simulink model "nmm2DFullBody"  (R2015b)
settings: Solver=ode23s  StartTime=0.0  StopTime=13  FixedStep=1e-3  MaxStep=ts_max  RelTol=1e-3  AbsTol=1e-4
InitFcn:
  | addpath('../lib');
  | addpath('./init_script');
  | nms_model_MechInit
  | nms_model_ControlInit
StopFcn:
  | mRFX = struct;
  | 
  | mRFX.RStance = DataFromModel.Data(:,2)
  | mRFX.RGRF_AP = DataFromModel.Data(:,24)
  | mRFX.RGRF_VT = DataFromModel.Data(:,22)
  | mRFX.RAnkleAngle = DataFromModel.Data(:,8)
  | mRFX.RKneeAngle = DataFromModel.Data(:,7)
  | mRFX.RHipAngle = DataFromModel.Data(:,6)
  | mRFX.RAnkleTorque = DataFromModel.Data(:,20)
  | mRFX.RKneeTorque = DataFromModel.Data(:,19)
  | mRFX.RHipTorque = DataFromModel.Data(:,18)
  | 
  | mRFX.RMuscleGLU = DataFromModel.Data(:,32)
  | mRFX.RMuscleHF = DataFromModel.Data(:,33)
  | mRFX.RMuscleHAM = DataFromModel.Data(:,34)
  | mRFX.RMuscleVAS = DataFromModel.Data(:,35)
  | mRFX.RMuscleGAS = DataFromModel.Data(:,36)
  | mRFX.RMuscleSOL = DataFromModel.Data(:,37)
  | mRFX.RMuscleTA = DataFromModel.Data(:,38)
  | 
  | mRFX.LStance = DataFromModel.Data(:,1)
  | mRFX.LGRF_AP = DataFromModel.Data(:,23)
  | mRFX.LGRF_VT = DataFromModel.Data(:,21)
  | mRFX.LAnkleAngle = DataFromModel.Data(:,5)
  | mRFX.LKneeAngle = DataFromModel.Data(:,4)
  | mRFX.LHipAngle = DataFromModel.Data(:,3)
  | mRFX.LAnkleTorque = DataFromModel.Data(:,17)
  | mRFX.LKneeTorque = DataFromModel.Data(:,16)
  | mRFX.LHipTorque = DataFromModel.Data(:,15)
  | 
  | mRFX.LMuscleGLU = DataFromModel.Data(:,25)
  | mRFX.LMuscleHF = DataFromModel.Data(:,26)
  | mRFX.LMuscleHAM = DataFromModel.Data(:,27)
  | mRFX.LMuscleVAS = DataFromModel.Data(:,28)
  | mRFX.LMuscleGAS = DataFromModel.Data(:,29)
  | mRFX.LMuscleSOL = DataFromModel.Data(:,30)
  | mRFX.LMuscleTA = DataFromModel.Data(:,31)
values from neighbouring files (symbols this model uses):
  c = load('struct_mRFX_HAM_symetric_feedback.mat')    [Ex2b.m]
undefined symbols (not defined in the file or in its folder): alphaFmGas, alphaFmGlu, alphaFmHam, alphaFmSol, alphaFmVas, alphaLceHam, alphaLceHfl, alphaLceTa, alphaLceTa1, Amp, amp_var, c_jointstop, D12_F, D12_S, D12_T, D13_F, D1G_F, D1G_HAT, D1G_S, D1G_T, DeltaThRef, eref, FmaxGAS, FmaxGLU, FmaxHAM, FmaxHFL, FmaxSOL, FmaxTA, FmaxVAS, freq, freq_var, GainDeltaTheta, GainGAS, GainGLU, GainHAM, GainHAMHFL, GainHFL, GainKneOverExt, GainSOL, GainSOLTA, GainTA, GainVAS, In_F, In_HAT, In_S, In_T, K, k_gx, k_gy, k_pressure, K_swing, LceOffsetHAM, LceOffsetHFL, LceOffsetTA, LongDelay, loptGAS, loptGLU, loptHAM, loptHFL, loptSOL ... (+82)
libraries: nmc x77, mblibv1 x60, simulink x33, simulink_extras x18
(part 3 of 8)

== system nmm2DFullBody/Body Mechanics Layer (from Geyer s 2010 model)/Left Heel Contact/Ground Friction Model ==
  note: Vertical Ground Stiction Model
  note: Horizontal Ground Friction Model
  dy [m] : Inport
  vy [m/s] : Inport  Port=2
  x [m] : Inport  Port=3
  vx [m/s] : Inport  Port=4
  Contact! : EnablePort  StatesWhenEnabling=reset
  Data Type Conversion : DataTypeConversion  OutDataTypeStr=double
  Friction Switch : Subsystem
  Gain3 : Gain  Gain=k_gy
  Gain4 : Gain  Gain=1/v_gy_max
  Logical Operator : Logic  Operator=NOT  AllPortsSameDT=off  OutDataTypeStr=boolean
  Mux1 : Mux  Inputs=2
  Sum1 : Sum
  X-Axis Kinetic Friction Model : Subsystem
  X-Axis Static Friction Model : Subsystem
  Y-Axis Ground Force : Fcn  Expr="- u(1)  *  (1-u(2)) * (u(2)<1)"
  Fy_Ground[N] : Outport  OutputWhenDisabled=reset  InitialOutput=0
      settings: AttributesFormatString=initial = '%<InitialOutput>'\nwhen disabled = '%<OutputWhenDisabled>'
  Fx_Friction [N] : Outport  Port=2  OutputWhenDisabled=reset  InitialOutput=0
      settings: AttributesFormatString=initial = '%<InitialOutput>'\nwhen\ndisabled\n'%<OutputWhenDisabled>'
  Stiction! : Outport  Port=3  OutputWhenDisabled=reset  InitialOutput=0
      settings: AttributesFormatString=initial = '%<InitialOutput>'\nwhen\ndisabled\n'%<OutputWhenDisabled>'
  wires:
  Gain4/1 -> Mux1/2
  Gain3/1 -> Mux1/1
  Mux1/1 -> Y-Axis Ground Force/1
  Data Type Conversion/1 -> Stiction!/1
  Logical Operator/1 -> X-Axis Kinetic Friction Model/Enable
  X-Axis Kinetic Friction Model/2(Stiction!) -> Friction Switch/2(Stick!)
  X-Axis Static Friction Model/2(Sliding!) -> Friction Switch/1(Slide!)
  Friction Switch/1(Stiction) -> Data Type Conversion/1, Logical Operator/1, X-Axis Static Friction Model/Enable
  Sum1/1 -> Fx_Friction [N]/1
  X-Axis Static Friction Model/1(F_Stick [N]) -> Sum1/1
  X-Axis Kinetic Friction Model/3(F_Slide [N]) -> Sum1/2
  X-Axis Kinetic Friction Model/1(posFP [m]) -> X-Axis Static Friction Model/4(posFP [m])
  vx [m/s]/1 -> X-Axis Kinetic Friction Model/2(vel [m/s]), X-Axis Static Friction Model/3(vel [m/s])
  x [m]/1 -> X-Axis Kinetic Friction Model/1(pos [m]), X-Axis Static Friction Model/2(pos [m])
  vy [m/s]/1 -> Gain4/1
  dy [m]/1 -> Gain3/1
  Y-Axis Ground Force/1 -> Fy_Ground[N]/1, X-Axis Kinetic Friction Model/3(F_Normal [N]), X-Axis Static Friction Model/1(F_Normal [N])

== system nmm2DFullBody/Body Mechanics Layer (from Geyer s 2010 model)/Right Ball Contact/Ground Friction Model ==
  note: Horizontal Ground Friction Model
  note: Vertical Ground Stiction Model
  dy [m] : Inport
  vy [m/s] : Inport  Port=2
  x [m] : Inport  Port=3
  vx [m/s] : Inport  Port=4
  Contact! : EnablePort  StatesWhenEnabling=reset
  Data Type Conversion : DataTypeConversion  OutDataTypeStr=double
  Friction Switch : Subsystem
  Gain3 : Gain  Gain=k_gy
  Gain4 : Gain  Gain=1/v_gy_max
  Logical Operator : Logic  Operator=NOT  AllPortsSameDT=off  OutDataTypeStr=boolean
  Mux1 : Mux  Inputs=2
  Sum1 : Sum
  X-Axis Kinetic Friction Model : Subsystem
  X-Axis Static Friction Model : Subsystem
  Y-Axis Ground Force : Fcn  Expr="- u(1)  *  (1-u(2)) * (u(2)<1)"
  Fy_Ground[N] : Outport  OutputWhenDisabled=reset  InitialOutput=0
      settings: AttributesFormatString=initial = '%<InitialOutput>'\nwhen disabled = '%<OutputWhenDisabled>'
  Fx_Friction [N] : Outport  Port=2  OutputWhenDisabled=reset  InitialOutput=0
      settings: AttributesFormatString=initial = '%<InitialOutput>'\nwhen\ndisabled\n'%<OutputWhenDisabled>'
  Stiction! : Outport  Port=3  OutputWhenDisabled=reset  InitialOutput=0
      settings: AttributesFormatString=initial = '%<InitialOutput>'\nwhen\ndisabled\n'%<OutputWhenDisabled>'
  wires:
  dy [m]/1 -> Gain3/1
  vy [m/s]/1 -> Gain4/1
  x [m]/1 -> X-Axis Static Friction Model/2(pos [m]), X-Axis Kinetic Friction Model/1(pos [m])
  vx [m/s]/1 -> X-Axis Static Friction Model/3(vel [m/s]), X-Axis Kinetic Friction Model/2(vel [m/s])
  X-Axis Kinetic Friction Model/1(posFP [m]) -> X-Axis Static Friction Model/4(posFP [m])
  X-Axis Kinetic Friction Model/3(F_Slide [N]) -> Sum1/2
  X-Axis Static Friction Model/1(F_Stick [N]) -> Sum1/1
  Sum1/1 -> Fx_Friction [N]/1
  Friction Switch/1(Stiction) -> X-Axis Static Friction Model/Enable, Logical Operator/1, Data Type Conversion/1
  X-Axis Static Friction Model/2(Sliding!) -> Friction Switch/1(Slide!)
  X-Axis Kinetic Friction Model/2(Stiction!) -> Friction Switch/2(Stick!)
  Logical Operator/1 -> X-Axis Kinetic Friction Model/Enable
  Data Type Conversion/1 -> Stiction!/1
  Mux1/1 -> Y-Axis Ground Force/1
  Gain3/1 -> Mux1/1
  Gain4/1 -> Mux1/2
  Y-Axis Ground Force/1 -> Fy_Ground[N]/1, X-Axis Static Friction Model/1(F_Normal [N]), X-Axis Kinetic Friction Model/3(F_Normal [N])

== system nmm2DFullBody/Body Mechanics Layer (from Geyer s 2010 model)/Right Heel Contact/Ground Friction Model ==
  note: Vertical Ground Stiction Model
  note: Horizontal Ground Friction Model
  dy [m] : Inport
  vy [m/s] : Inport  Port=2
  x [m] : Inport  Port=3
  vx [m/s] : Inport  Port=4
  Contact! : EnablePort  StatesWhenEnabling=reset
  Data Type Conversion : DataTypeConversion  OutDataTypeStr=double
  Friction Switch : Subsystem
  Gain3 : Gain  Gain=k_gy
  Gain4 : Gain  Gain=1/v_gy_max
  Logical Operator : Logic  Operator=NOT  AllPortsSameDT=off  OutDataTypeStr=boolean
  Mux1 : Mux  Inputs=2
  Sum1 : Sum
  X-Axis Kinetic Friction Model : Subsystem
  X-Axis Static Friction Model : Subsystem
  Y-Axis Ground Force : Fcn  Expr="- u(1)  *  (1-u(2)) * (u(2)<1)"
  Fy_Ground[N] : Outport  OutputWhenDisabled=reset  InitialOutput=0
      settings: AttributesFormatString=initial = '%<InitialOutput>'\nwhen disabled = '%<OutputWhenDisabled>'
  Fx_Friction [N] : Outport  Port=2  OutputWhenDisabled=reset  InitialOutput=0
      settings: AttributesFormatString=initial = '%<InitialOutput>'\nwhen\ndisabled\n'%<OutputWhenDisabled>'
  Stiction! : Outport  Port=3  OutputWhenDisabled=reset  InitialOutput=0
      settings: AttributesFormatString=initial = '%<InitialOutput>'\nwhen\ndisabled\n'%<OutputWhenDisabled>'
  wires:
  Gain4/1 -> Mux1/2
  Gain3/1 -> Mux1/1
  Mux1/1 -> Y-Axis Ground Force/1
  Data Type Conversion/1 -> Stiction!/1
  Logical Operator/1 -> X-Axis Kinetic Friction Model/Enable
  X-Axis Kinetic Friction Model/2(Stiction!) -> Friction Switch/2(Stick!)
  X-Axis Static Friction Model/2(Sliding!) -> Friction Switch/1(Slide!)
  Friction Switch/1(Stiction) -> Data Type Conversion/1, Logical Operator/1, X-Axis Static Friction Model/Enable
  Sum1/1 -> Fx_Friction [N]/1
  X-Axis Static Friction Model/1(F_Stick [N]) -> Sum1/1
  X-Axis Kinetic Friction Model/3(F_Slide [N]) -> Sum1/2
  X-Axis Kinetic Friction Model/1(posFP [m]) -> X-Axis Static Friction Model/4(posFP [m])
  vx [m/s]/1 -> X-Axis Kinetic Friction Model/2(vel [m/s]), X-Axis Static Friction Model/3(vel [m/s])
  x [m]/1 -> X-Axis Kinetic Friction Model/1(pos [m]), X-Axis Static Friction Model/2(pos [m])
  vy [m/s]/1 -> Gain4/1
  dy [m]/1 -> Gain3/1
  Y-Axis Ground Force/1 -> Fy_Ground[N]/1, X-Axis Kinetic Friction Model/3(F_Normal [N]), X-Axis Static Friction Model/1(F_Normal [N])

== system nmm2DFullBody/Full Body Control (created using the nmc library)/Left Side/AnkleJoint left ==
  note: Ankle Joint
  phidphiAnkle : Inport
  PreTauAnkle : Inport  Port=2
  " Ankle Joint Limits" : Subsystem
  Demux : Demux  Outputs=2
  GotoDisabler_Component : nmc/GotoDisabler_Component  GotoTag=DisableNMC_JointLimits
  Sum : Sum  Inputs=|++
  Sum of Elements : Sum  Inputs=+
  TauAnkle : Outport
  wires:
  Demux/1 -> " Ankle Joint Limits"/1(phi [rad])
  Demux/2 -> " Ankle Joint Limits"/2(dphi [rad/s])
  PreTauAnkle/1 -> Sum of Elements/1
  phidphiAnkle/1 -> Demux/1
  " Ankle Joint Limits"/1(M_stop [Nm]) -> GotoDisabler_Component/1
  Sum/1 -> TauAnkle/1
  Sum of Elements/1 -> Sum/2
  GotoDisabler_Component/1 -> Sum/1

== system nmm2DFullBody/Full Body Control (created using the nmc library)/Left Side/GAS Muscle ==
  note: GAS Muscle
  phiKnee : Inport
  phiAnkle : Inport  Port=2
  StanceSwing : Inport  Port=3
  "GAS Actuation " : Subsystem
  GAS Control : Subsystem
  LOG_GasAnkle : Concatenate  NumInputs=1
  LOG_TauGasKnee : Concatenate  NumInputs=1
  StimGAS : ToWorkspace  VariableName=StimGASL  SaveFormat=Timeseries  SampleTime=-1
  TauGasKnee : Outport
  TauGasAnkle : Outport  Port=2
  wires:
  LOG_GasAnkle/1 -> TauGasAnkle/1
  LOG_TauGasKnee/1 -> TauGasKnee/1
  phiAnkle/1 -> "GAS Actuation "/2(phiAnkle)
  "GAS Actuation "/1(TauGasKnee) -> LOG_TauGasKnee/1
  "GAS Actuation "/2(TauGasAnkle) -> LOG_GasAnkle/1
  "GAS Actuation "/3(FmGas) -> GAS Control/1(FmGAS)
  StanceSwing/1 -> GAS Control/2(StanceSwing)
  phiKnee/1 -> "GAS Actuation "/1(phiKnee)
  GAS Control/1(StimGAS) -> StimGAS/1, "GAS Actuation "/3(StimGas)

== system nmm2DFullBody/Full Body Control (created using the nmc library)/Left Side/GLU Muscle ==
  note: GLU Muscle
  phiHip : Inport
  CLdxThigh : Inport  Port=2
  OLonCL : Inport  Port=3
  StanceSwing : Inport  Port=4
  GLU Actuation : Subsystem
  GLU Control : Subsystem
  LOG_TauGlu : Concatenate  NumInputs=1
  StimGLU : ToWorkspace  VariableName=StimGLU1  SaveFormat=Timeseries  SampleTime=-1
  TauGlu : Outport
  wires:
  LOG_TauGlu/1 -> TauGlu/1
  GLU Control/1(StimGlu) -> GLU Actuation/2(StimGlu), StimGLU/1
  GLU Actuation/2(FmGlu) -> GLU Control/1(FmGlu)
  OLonCL/1 -> GLU Control/5(OLonCL)
  [ThetaDelayed] -> GLU Control/2(Theta)
  [dThetaDelayed] -> GLU Control/3(dTheta)
  phiHip/1 -> GLU Actuation/1(phiHip)
  CLdxThigh/1 -> GLU Control/4(CLdxThigh)
  StanceSwing/1 -> GLU Control/6(StanceSwing)
  GLU Actuation/1(TauGlu) -> LOG_TauGlu/1

== system nmm2DFullBody/Full Body Control (created using the nmc library)/Left Side/HFL&HAM Muscles ==
  note: HFL&HAM Muscles
  phiHip : Inport
  phiKnee : Inport  Port=2
  CLdxThigh : Inport  Port=3
  OLonCL : Inport  Port=4
  StanceSwing : Inport  Port=5
  "HAM Actuation " : Subsystem
  HFL Actuation : Subsystem
  HFL&HAM Control : Subsystem
  LOG_TauHFL : Concatenate  NumInputs=1
  LOG_TauHamHip : Concatenate  NumInputs=1
  LOG_TauHamKnee : Concatenate  NumInputs=1
  StimHAM : ToWorkspace  VariableName=StimHAM  SaveFormat=Timeseries  SampleTime=-1
  StimHFL : ToWorkspace  VariableName=StimHFL  SaveFormat=Timeseries  SampleTime=-1
  TauHFL : Outport
  TauHamHip : Outport  Port=2
  TauHamKnee : Outport  Port=3
  wires:
  LOG_TauHamKnee/1 -> TauHamKnee/1
  LOG_TauHamHip/1 -> TauHamHip/1
  LOG_TauHFL/1 -> TauHFL/1
  HFL&HAM Control/2(StimHAM) -> StimHAM/1, "HAM Actuation "/3(StimHam)
  StanceSwing/1 -> HFL&HAM Control/8(StanceSwing)
  [dThetaDelayed] -> HFL&HAM Control/5(dTheta)
  [ThetaDelayed] -> HFL&HAM Control/4(Theta)
  phiKnee/1 -> "HAM Actuation "/2(phiKnee)
  HFL Actuation/1(TauHFL) -> LOG_TauHFL/1
  CLdxThigh/1 -> HFL&HAM Control/6(CLdxThigh)
  "HAM Actuation "/2(TauHamKnee) -> LOG_TauHamKnee/1
  phiHip/1 -> "HAM Actuation "/1(phiHip), HFL Actuation/1(phiHip)
  "HAM Actuation "/1(TauHamHip) -> LOG_TauHamHip/1
  OLonCL/1 -> HFL&HAM Control/7(OLonCL)
  HFL Actuation/2(LceHFL) -> HFL&HAM Control/1(LceHFL)
  "HAM Actuation "/4(FmHam) -> HFL&HAM Control/3(FmHam)
  "HAM Actuation "/3(LceHam) -> HFL&HAM Control/2(LceHam)
  HFL&HAM Control/1(StimHFL) -> StimHFL/1, HFL Actuation/2(StimHFL)

== system nmm2DFullBody/Full Body Control (created using the nmc library)/Left Side/HipJoint left ==
  note: Hip Joint
  phidphiHip : Inport
  PreTauHip : Inport  Port=2
  Demux2 : Demux  Outputs=2
  GotoDisabler_Component : nmc/GotoDisabler_Component  GotoTag=DisableNMC_JointLimits
  Hip Joint Limits : Subsystem
  Sum of Elements : Sum  Inputs=+
  Sum16 : Sum  Inputs=|++
  TauHip : Outport
  wires:
  phidphiHip/1 -> Demux2/1
  Demux2/1 -> Hip Joint Limits/1(phi [rad])
  Demux2/2 -> Hip Joint Limits/2(dphi [rad/s])
  Sum16/1 -> TauHip/1
  PreTauHip/1 -> Sum of Elements/1
  Sum of Elements/1 -> Sum16/2
  Hip Joint Limits/1(M_stop [Nm]) -> GotoDisabler_Component/1
  GotoDisabler_Component/1 -> Sum16/1

== system nmm2DFullBody/Full Body Control (created using the nmc library)/Left Side/KneeJoint left ==
  note: Knee Joint
  phidphiKnee : Inport
  PreTauKnee : Inport  Port=2
  Demux1 : Demux  Outputs=2
  Gain : Gain  Gain=-1
  GotoDisabler_Component : nmc/GotoDisabler_Component  GotoTag=DisableNMC_JointLimits
  Knee Joint Limits : Subsystem
  Sum : Sum  Inputs=|++
  Sum of Elements : Sum  Inputs=+
  TauKnee : Outport
  wires:
  Demux1/1 -> Knee Joint Limits/1(phi [rad])
  Demux1/2 -> Knee Joint Limits/2(dphi [rad/s])
  phidphiKnee/1 -> Demux1/1
  Sum/1 -> TauKnee/1
  PreTauKnee/1 -> Sum of Elements/1
  Sum of Elements/1 -> Gain/1
  Gain/1 -> Sum/2
  Knee Joint Limits/1(M_stop [Nm]) -> GotoDisabler_Component/1
  GotoDisabler_Component/1 -> Sum/1

== system nmm2DFullBody/Full Body Control (created using the nmc library)/Left Side/SOL&TA Muscles ==
  note: SOL&TA Muscles
  phiAnkle : Inport
  StanceSwing : Inport  Port=2
  LOG_StimSOL : Concatenate  NumInputs=1
  LOG_StimTA : Concatenate  NumInputs=1
  LOG_TauSOL : Concatenate  NumInputs=1
  LOG_TauTA : Concatenate  NumInputs=1
  SOL Actuation : Subsystem
  SOL&TA Control : Subsystem
  StimSOL : ToWorkspace  VariableName=StimSOLL  SaveFormat=Timeseries  SampleTime=-1
  StimTA : ToWorkspace  VariableName=StimTAL  SaveFormat=Timeseries  SampleTime=-1
  TA Actuation : Subsystem
  TauTA : Outport
  TauSOL : Outport  Port=2
  wires:
  LOG_StimSOL/1 -> StimSOL/1, SOL Actuation/2(StimSOL)
  LOG_StimTA/1 -> TA Actuation/2(StimTA), StimTA/1
  LOG_TauSOL/1 -> TauSOL/1
  LOG_TauTA/1 -> TauTA/1
  TA Actuation/2(TauTa) -> LOG_TauTA/1
  phiAnkle/1 -> SOL Actuation/1(phiAnkle), TA Actuation/1(phiAnkle)
  TA Actuation/1(LceTA) -> SOL&TA Control/1(LceTA)
  StanceSwing/1 -> SOL&TA Control/3(StanceSwing)
  SOL&TA Control/1(StimTA) -> LOG_StimTA/1
  SOL Actuation/1(TauSOL) -> LOG_TauSOL/1
  SOL Actuation/2(FmSOL) -> SOL&TA Control/2(FmSOL)
  SOL&TA Control/2(StimSOL) -> LOG_StimSOL/1

== system nmm2DFullBody/Full Body Control (created using the nmc library)/Left Side/VAS Muscle ==
  note: VAS Muscle
  phiKnee : Inport
  OLdxThigh : Inport  Port=2
  OLonCL : Inport  Port=3
  CLKneeState : Inport  Port=4
  StanceSwing : Inport  Port=5
  LOG_TauVas : Concatenate  NumInputs=1
  StimVAS : ToWorkspace  VariableName=StimVAS  SaveFormat=Timeseries  SampleTime=-1
  "VAS Actuation " : Subsystem
  VAS Control : Subsystem
  TauVas : Outport
  wires:
  LOG_TauVas/1 -> TauVas/1
  VAS Control/1(StimVAS) -> StimVAS/1, "VAS Actuation "/2(StimVas)
  "VAS Actuation "/2(FmVas) -> VAS Control/1(FmVAS)
  "VAS Actuation "/1(TauVas) -> LOG_TauVas/1
  OLonCL/1 -> VAS Control/3(OLonCL)
  StanceSwing/1 -> VAS Control/5(StanceSwing)
  OLdxThigh/1 -> VAS Control/2(OLdxThigh)
  phiKnee/1 -> "VAS Actuation "/1(phiKnee)
  CLKneeState/1 -> VAS Control/4(CLKneeState)

== system nmm2DFullBody/Full Body Control (created using the nmc library)/Right Side/GAS Muscle ==
  note: GAS Muscle
  phiKnee : Inport
  phiAnkle : Inport  Port=2
  StanceSwing : Inport  Port=3
  "GAS Actuation " : Subsystem
  GAS Control : Subsystem
  LOG_GasAnkle : Concatenate  NumInputs=1
  LOG_TauGasKnee : Concatenate  NumInputs=1
  StimGAS : ToWorkspace  VariableName=StimGASR  SaveFormat=Timeseries  SampleTime=-1
  TauGasKnee : Outport
  TauGasAnkle : Outport  Port=2
  wires:
  LOG_GasAnkle/1 -> TauGasAnkle/1
  LOG_TauGasKnee/1 -> TauGasKnee/1
  phiAnkle/1 -> "GAS Actuation "/2(phiAnkle)
  "GAS Actuation "/1(TauGasKnee) -> LOG_TauGasKnee/1
  "GAS Actuation "/2(TauGasAnkle) -> LOG_GasAnkle/1
  "GAS Actuation "/3(FmGas) -> GAS Control/1(FmGAS)
  StanceSwing/1 -> GAS Control/2(StanceSwing)
  phiKnee/1 -> "GAS Actuation "/1(phiKnee)
  GAS Control/1(StimGAS) -> StimGAS/1, "GAS Actuation "/3(StimGas)

== system nmm2DFullBody/Full Body Control (created using the nmc library)/Right Side/GLU Muscle ==
  note: GLU Muscle
  phiHip : Inport
  CLdxThigh : Inport  Port=2
  OLonCL : Inport  Port=3
  StanceSwing : Inport  Port=4
  GLU Actuation : Subsystem
  GLU Control : Subsystem
  LOG_TauGlu : Concatenate  NumInputs=1
  StimGLU : ToWorkspace  VariableName=StimGLUR  SaveFormat=Timeseries  SampleTime=-1
  TauGlu : Outport
  wires:
  LOG_TauGlu/1 -> TauGlu/1
  GLU Control/1(StimGlu) -> GLU Actuation/2(StimGlu), StimGLU/1
  GLU Actuation/2(FmGlu) -> GLU Control/1(FmGlu)
  OLonCL/1 -> GLU Control/5(OLonCL)
  [ThetaDelayed] -> GLU Control/2(Theta)
  [dThetaDelayed] -> GLU Control/3(dTheta)
  phiHip/1 -> GLU Actuation/1(phiHip)
  CLdxThigh/1 -> GLU Control/4(CLdxThigh)
  StanceSwing/1 -> GLU Control/6(StanceSwing)
  GLU Actuation/1(TauGlu) -> LOG_TauGlu/1

== system nmm2DFullBody/Full Body Control (created using the nmc library)/Right Side/HFL&HAM Muscles ==
  note: HFL&HAM Muscles
  phiHip : Inport
  phiKnee : Inport  Port=2
  CLdxThigh : Inport  Port=3
  OLonCL : Inport  Port=4
  StanceSwing : Inport  Port=5
  "HAM Actuation " : Subsystem
  HFL Actuation : Subsystem
  HFL&HAM Control : Subsystem
  LOG_TauHFL : Concatenate  NumInputs=1
  LOG_TauHamHip : Concatenate  NumInputs=1
  LOG_TauHamKnee : Concatenate  NumInputs=1
  StimHAM : ToWorkspace  VariableName=StimHAMR  SaveFormat=Timeseries  SampleTime=-1
  StimHFL : ToWorkspace  VariableName=StimHFLR  SaveFormat=Timeseries  SampleTime=-1
  TauHFL : Outport
  TauHamHip : Outport  Port=2
  TauHamKnee : Outport  Port=3
  wires:
  LOG_TauHamKnee/1 -> TauHamKnee/1
  LOG_TauHamHip/1 -> TauHamHip/1
  LOG_TauHFL/1 -> TauHFL/1
  HFL&HAM Control/2(StimHAM) -> StimHAM/1, "HAM Actuation "/3(StimHam)
  StanceSwing/1 -> HFL&HAM Control/8(StanceSwing)
  [dThetaDelayed] -> HFL&HAM Control/5(dTheta)
  [ThetaDelayed] -> HFL&HAM Control/4(Theta)
  phiKnee/1 -> "HAM Actuation "/2(phiKnee)
  HFL Actuation/1(TauHFL) -> LOG_TauHFL/1
  CLdxThigh/1 -> HFL&HAM Control/6(CLdxThigh)
  "HAM Actuation "/2(TauHamKnee) -> LOG_TauHamKnee/1
  phiHip/1 -> "HAM Actuation "/1(phiHip), HFL Actuation/1(phiHip)
  "HAM Actuation "/1(TauHamHip) -> LOG_TauHamHip/1
  OLonCL/1 -> HFL&HAM Control/7(OLonCL)
  HFL Actuation/2(LceHFL) -> HFL&HAM Control/1(LceHFL)
  "HAM Actuation "/4(FmHam) -> HFL&HAM Control/3(FmHam)
  "HAM Actuation "/3(LceHam) -> HFL&HAM Control/2(LceHam)
  HFL&HAM Control/1(StimHFL) -> StimHFL/1, HFL Actuation/2(StimHFL)

== system nmm2DFullBody/Full Body Control (created using the nmc library)/Right Side/SOL&TA Muscles ==
  note: SOL&TA Muscles
  phiAnkle : Inport
  StanceSwing : Inport  Port=2
  LOG_StimSOL : Concatenate  NumInputs=1
  LOG_StimTA : Concatenate  NumInputs=1
  LOG_TauSOL : Concatenate  NumInputs=1
  LOG_TauTA : Concatenate  NumInputs=1
  SOL Actuation : Subsystem
  SOL&TA Control : Subsystem
  StimSOL : ToWorkspace  VariableName=StimSOLR  SaveFormat=Timeseries  SampleTime=-1
  StimTA : ToWorkspace  VariableName=StimTAR  SaveFormat=Timeseries  SampleTime=-1
  TA Actuation : Subsystem
  TauTA : Outport
  TauSOL : Outport  Port=2
  wires:
  LOG_StimSOL/1 -> StimSOL/1, SOL Actuation/2(StimSOL)
  LOG_StimTA/1 -> TA Actuation/2(StimTA), StimTA/1
  LOG_TauSOL/1 -> TauSOL/1
  LOG_TauTA/1 -> TauTA/1
  TA Actuation/2(TauTa) -> LOG_TauTA/1
  phiAnkle/1 -> SOL Actuation/1(phiAnkle), TA Actuation/1(phiAnkle)
  TA Actuation/1(LceTA) -> SOL&TA Control/1(LceTA)
  StanceSwing/1 -> SOL&TA Control/3(StanceSwing)
  SOL&TA Control/1(StimTA) -> LOG_StimTA/1
  SOL Actuation/1(TauSOL) -> LOG_TauSOL/1
  SOL Actuation/2(FmSOL) -> SOL&TA Control/2(FmSOL)
  SOL&TA Control/2(StimSOL) -> LOG_StimSOL/1

== system nmm2DFullBody/Full Body Control (created using the nmc library)/Right Side/VAS Muscle ==
  note: VAS Muscle
  phiKnee : Inport
  OLdxThigh : Inport  Port=2
  OLonCL : Inport  Port=3
  CLKneeState : Inport  Port=4
  StanceSwing : Inport  Port=5
  LOG_TauVas : Concatenate  NumInputs=1
  StimVAS : ToWorkspace  VariableName=StimVASR  SaveFormat=Timeseries  SampleTime=-1
  "VAS Actuation " : Subsystem
  VAS Control : Subsystem
  TauVas : Outport
  wires:
  LOG_TauVas/1 -> TauVas/1
  VAS Control/1(StimVAS) -> StimVAS/1, "VAS Actuation "/2(StimVas)
  "VAS Actuation "/2(FmVas) -> VAS Control/1(FmVAS)
  "VAS Actuation "/1(TauVas) -> LOG_TauVas/1
  OLonCL/1 -> VAS Control/3(OLonCL)
  StanceSwing/1 -> VAS Control/5(StanceSwing)
  OLdxThigh/1 -> VAS Control/2(OLdxThigh)
  phiKnee/1 -> "VAS Actuation "/1(phiKnee)
  CLKneeState/1 -> VAS Control/4(CLKneeState)

== system nmm2DFullBody/Full Body Control (created using the nmc library)/Subsystem/Parameter variation ==
  Alpha variation : Subsystem  Commented=on
  Amplitude Variation : Subsystem  Commented=on
  Freq variation : Subsystem  Commented=on

== system nmm2DFullBody/Body Mechanics Layer (from Geyer s 2010 model)/Left Ball Contact/Ground Friction Model/Friction Switch ==
  note: Static/Kinetic Friction Switch
  Slide! : Inport
  Stick! : Inport  Port=2
  Memory : Memory
  S-R Flip-Flop : simulink_extras/Flip Flops/S-R Flip-Flop  initial_condition=1
  Terminator : Terminator
  Stiction : Outport
  wires:
  S-R Flip-Flop/1 -> Memory/1
  S-R Flip-Flop/2 -> Terminator/1
  Stick!/1 -> S-R Flip-Flop/1
  Slide!/1 -> S-R Flip-Flop/2
  Memory/1 -> Stiction/1

== system nmm2DFullBody/Body Mechanics Layer (from Geyer s 2010 model)/Left Ball Contact/Ground Friction Model/X-Axis Kinetic Friction Model ==
  note: Kinetic Friction Model
  note: Footpoint Determiner
  note: Sliding Limit Detector
  pos [m] : Inport
  vel [m/s] : Inport  Port=2
  F_Normal [N] : Inport  Port=3
  Enable : EnablePort  StatesWhenEnabling=reset  ZeroCross=off
  Abs : Abs
  Constant : Constant  Value=vLimit
  FixPt Relational Operator : RelationalOperator  Operator=>  OutDataTypeStr=boolean  ZeroCross=off
  Memory : Memory
  Negative : simulink/Logic and Bit Operations/Compare To Zero  relop=<  OutDataTypeStr=boolean
  Product : Product  RndMeth=Zero
  Sign1 : Signum
  Sum : Sum  Inputs=|+-
  reverse : Gain  Gain=-1
  sliding friction coefficient : Gain  Gain=mu_slide
  posFP [m] : Outport  InitialOutput=0
      settings: AttributesFormatString=initial = '%<InitialOutput>'\nwhen disabled = '%<OutputWhenDisabled>'
  Stiction! : Outport  Port=2  OutputWhenDisabled=reset  InitialOutput=0
      settings: AttributesFormatString=initial = '%<InitialOutput>'\nwhen disabled = '%<OutputWhenDisabled>'
  F_Slide [N] : Outport  Port=3  OutputWhenDisabled=reset  InitialOutput=0
      settings: AttributesFormatString=initial = '%<InitialOutput>'\nwhen disabled = '%<OutputWhenDisabled>'
  wires:
  reverse/1 -> Product/1
  F_Normal [N]/1 -> sliding friction coefficient/1
  vel [m/s]/1 -> Sign1/1, Abs/1
  pos [m]/1 -> posFP [m]/1
  Product/1 -> F_Slide [N]/1
  sliding friction coefficient/1 -> Product/2
  Sign1/1 -> reverse/1
  FixPt Relational Operator/1 -> Stiction!/1
  Memory/1 -> FixPt Relational Operator/2
  Negative/1 -> FixPt Relational Operator/1, Memory/1
  Abs/1 -> Sum/1
  Sum/1 -> Negative/1
  Constant/1 -> Sum/2

== system nmm2DFullBody/Body Mechanics Layer (from Geyer s 2010 model)/Left Ball Contact/Ground Friction Model/X-Axis Static Friction Model ==
  note: Stiction Limit Detector
  note: Static Friction Model
  note: Zero multiplication prevents
      | horizontal friction model from
      | oscillating between static and kinetic
      | friction when the vertical force is zero but
      | the ground level is not yet reached
      | in the upward motion
  F_Normal [N] : Inport
  pos [m] : Inport  Port=2
  vel [m/s] : Inport  Port=3
  posFP [m] : Inport  Port=4
  Enable : EnablePort  StatesWhenEnabling=reset  ZeroCross=off
  Abs : Abs
  Abs. : Abs
  Check Vertical Friction : Product  RndMeth=Zero
  FixPt Relational Operator : RelationalOperator  Operator=>  OutDataTypeStr=boolean  ZeroCross=off
  Gain3 : Gain  Gain=k_gx
  Gain4 : Gain  Gain=1/v_gx_max
  Memory : Memory
  Mux1 : Mux  Inputs=2
  Positive : simulink/Logic and Bit Operations/Compare To Zero  relop=>  OutDataTypeStr=boolean
  Positive1 : simulink/Logic and Bit Operations/Compare To Zero  relop=>  OutDataTypeStr=boolean
  Sum : Sum  Inputs=-+
  Sum2 : Sum  Inputs=-+|
  X-Axis Stiction Force : Fcn  Expr=-u(1) * (1+sgn(u(1))*u(2))
  stiction limit force : Gain  Gain=mu_stick
  F_Stick [N] : Outport  OutputWhenDisabled=reset  InitialOutput=0
      settings: AttributesFormatString=when disabled: %<OutputWhenDisabled>\ninitial: %<InitialOutput>
  Sliding! : Outport  Port=2  OutputWhenDisabled=reset  InitialOutput=0
      settings: AttributesFormatString=when disabled: %<OutputWhenDisabled>\ninitial: %<InitialOutput>
  wires:
  F_Normal [N]/1 -> stiction limit force/1, Positive1/1
  Sum2/1 -> Gain3/1  "dx"
  pos [m]/1 -> Sum2/2
  posFP [m]/1 -> Sum2/1
  vel [m/s]/1 -> Gain4/1
  Sum/1 -> Positive/1
  Memory/1 -> FixPt Relational Operator/2
  Positive/1 -> FixPt Relational Operator/1, Memory/1
  Abs./1 -> Sum/2
  Mux1/1 -> X-Axis Stiction Force/1
  Gain3/1 -> Mux1/1
  Gain4/1 -> Mux1/2
  FixPt Relational Operator/1 -> Sliding!/1
  Abs/1 -> Sum/1
  stiction limit force/1 -> Abs/1
  X-Axis Stiction Force/1 -> Check Vertical Friction/1
  Positive1/1 -> Check Vertical Friction/2
  Check Vertical Friction/1 -> F_Stick [N]/1, Abs./1

== system nmm2DFullBody/Body Mechanics Layer (from Geyer s 2010 model)/Left Heel Contact/Ground Friction Model/Friction Switch ==
  note: Static/Kinetic Friction Switch
  Slide! : Inport
  Stick! : Inport  Port=2
  Memory : Memory
  S-R Flip-Flop : simulink_extras/Flip Flops/S-R Flip-Flop  initial_condition=1
  Terminator : Terminator
  Stiction : Outport
  wires:
  Memory/1 -> Stiction/1
  Slide!/1 -> S-R Flip-Flop/2
  Stick!/1 -> S-R Flip-Flop/1
  S-R Flip-Flop/2 -> Terminator/1
  S-R Flip-Flop/1 -> Memory/1

== system nmm2DFullBody/Body Mechanics Layer (from Geyer s 2010 model)/Left Heel Contact/Ground Friction Model/X-Axis Kinetic Friction Model ==
  note: Sliding Limit Detector
  note: Footpoint Determiner
  note: Kinetic Friction Model
  pos [m] : Inport
  vel [m/s] : Inport  Port=2
  F_Normal [N] : Inport  Port=3
  Enable : EnablePort  StatesWhenEnabling=reset  ZeroCross=off
  Abs : Abs
  Constant : Constant  Value=vLimit
  FixPt Relational Operator : RelationalOperator  Operator=>  OutDataTypeStr=boolean  ZeroCross=off
  Memory : Memory
  Negative : simulink/Logic and Bit Operations/Compare To Zero  relop=<  OutDataTypeStr=boolean
  Product : Product  RndMeth=Zero
  Sign1 : Signum
  Sum : Sum  Inputs=|+-
  reverse : Gain  Gain=-1
  sliding friction coefficient : Gain  Gain=mu_slide
  posFP [m] : Outport  InitialOutput=0
      settings: AttributesFormatString=initial = '%<InitialOutput>'\nwhen disabled = '%<OutputWhenDisabled>'
  Stiction! : Outport  Port=2  OutputWhenDisabled=reset  InitialOutput=0
      settings: AttributesFormatString=initial = '%<InitialOutput>'\nwhen disabled = '%<OutputWhenDisabled>'
  F_Slide [N] : Outport  Port=3  OutputWhenDisabled=reset  InitialOutput=0
      settings: AttributesFormatString=initial = '%<InitialOutput>'\nwhen disabled = '%<OutputWhenDisabled>'
  wires:
  Constant/1 -> Sum/2
  Sum/1 -> Negative/1
  Abs/1 -> Sum/1
  Negative/1 -> Memory/1, FixPt Relational Operator/1
  Memory/1 -> FixPt Relational Operator/2
  FixPt Relational Operator/1 -> Stiction!/1
  Sign1/1 -> reverse/1
  sliding friction coefficient/1 -> Product/2
  Product/1 -> F_Slide [N]/1
  pos [m]/1 -> posFP [m]/1
  vel [m/s]/1 -> Abs/1, Sign1/1
  F_Normal [N]/1 -> sliding friction coefficient/1
  reverse/1 -> Product/1

== system nmm2DFullBody/Body Mechanics Layer (from Geyer s 2010 model)/Left Heel Contact/Ground Friction Model/X-Axis Static Friction Model ==
  note: Static Friction Model
  note: Stiction Limit Detector
  note: Zero multiplication prevents
      | horizontal friction model from
      | oscillating between static and kinetic
      | friction when the vertical force is zero but
      | the ground level is not yet reached
      | in the upward motion
  F_Normal [N] : Inport
  pos [m] : Inport  Port=2
  vel [m/s] : Inport  Port=3
  posFP [m] : Inport  Port=4
  Enable : EnablePort  StatesWhenEnabling=reset  ZeroCross=off
  Abs : Abs
  Abs. : Abs
  Check Vertical Friction : Product  RndMeth=Zero
  FixPt Relational Operator : RelationalOperator  Operator=>  OutDataTypeStr=boolean  ZeroCross=off
  Gain3 : Gain  Gain=k_gx
  Gain4 : Gain  Gain=1/v_gx_max
  Memory : Memory
  Mux1 : Mux  Inputs=2
  Positive : simulink/Logic and Bit Operations/Compare To Zero  relop=>  OutDataTypeStr=boolean
  Positive1 : simulink/Logic and Bit Operations/Compare To Zero  relop=>  OutDataTypeStr=boolean
  Sum : Sum  Inputs=-+
  Sum2 : Sum  Inputs=-+|
  X-Axis Stiction Force : Fcn  Expr=-u(1) * (1+sgn(u(1))*u(2))
  stiction limit force : Gain  Gain=mu_stick
  F_Stick [N] : Outport  OutputWhenDisabled=reset  InitialOutput=0
      settings: AttributesFormatString=when disabled: %<OutputWhenDisabled>\ninitial: %<InitialOutput>
  Sliding! : Outport  Port=2  OutputWhenDisabled=reset  InitialOutput=0
      settings: AttributesFormatString=when disabled: %<OutputWhenDisabled>\ninitial: %<InitialOutput>
  wires:
  F_Normal [N]/1 -> stiction limit force/1, Positive1/1
  Sum2/1 -> Gain3/1  "dx"
  pos [m]/1 -> Sum2/2
  posFP [m]/1 -> Sum2/1
  vel [m/s]/1 -> Gain4/1
  Sum/1 -> Positive/1
  Memory/1 -> FixPt Relational Operator/2
  Positive/1 -> FixPt Relational Operator/1, Memory/1
  Abs./1 -> Sum/2
  Mux1/1 -> X-Axis Stiction Force/1
  Gain3/1 -> Mux1/1
  Gain4/1 -> Mux1/2
  FixPt Relational Operator/1 -> Sliding!/1
  Abs/1 -> Sum/1
  stiction limit force/1 -> Abs/1
  X-Axis Stiction Force/1 -> Check Vertical Friction/1
  Positive1/1 -> Check Vertical Friction/2
  Check Vertical Friction/1 -> F_Stick [N]/1, Abs./1

== system nmm2DFullBody/Body Mechanics Layer (from Geyer s 2010 model)/Right Ball Contact/Ground Friction Model/Friction Switch ==
  note: Static/Kinetic Friction Switch
  Slide! : Inport
  Stick! : Inport  Port=2
  Memory : Memory
  S-R Flip-Flop : simulink_extras/Flip Flops/S-R Flip-Flop  initial_condition=1
  Terminator : Terminator
  Stiction : Outport
  wires:
  S-R Flip-Flop/1 -> Memory/1
  S-R Flip-Flop/2 -> Terminator/1
  Stick!/1 -> S-R Flip-Flop/1
  Slide!/1 -> S-R Flip-Flop/2
  Memory/1 -> Stiction/1

== system nmm2DFullBody/Body Mechanics Layer (from Geyer s 2010 model)/Right Ball Contact/Ground Friction Model/X-Axis Kinetic Friction Model ==
  note: Kinetic Friction Model
  note: Footpoint Determiner
  note: Sliding Limit Detector
  pos [m] : Inport
  vel [m/s] : Inport  Port=2
  F_Normal [N] : Inport  Port=3
  Enable : EnablePort  StatesWhenEnabling=reset  ZeroCross=off
  Abs : Abs
  Constant : Constant  Value=vLimit
  FixPt Relational Operator : RelationalOperator  Operator=>  OutDataTypeStr=boolean  ZeroCross=off
  Memory : Memory
  Negative : simulink/Logic and Bit Operations/Compare To Zero  relop=<  OutDataTypeStr=boolean
  Product : Product  RndMeth=Zero
  Sign1 : Signum
  Sum : Sum  Inputs=|+-
  reverse : Gain  Gain=-1
  sliding friction coefficient : Gain  Gain=mu_slide
  posFP [m] : Outport  InitialOutput=0
      settings: AttributesFormatString=initial = '%<InitialOutput>'\nwhen disabled = '%<OutputWhenDisabled>'
  Stiction! : Outport  Port=2  OutputWhenDisabled=reset  InitialOutput=0
      settings: AttributesFormatString=initial = '%<InitialOutput>'\nwhen disabled = '%<OutputWhenDisabled>'
  F_Slide [N] : Outport  Port=3  OutputWhenDisabled=reset  InitialOutput=0
      settings: AttributesFormatString=initial = '%<InitialOutput>'\nwhen disabled = '%<OutputWhenDisabled>'
  wires:
  reverse/1 -> Product/1
  F_Normal [N]/1 -> sliding friction coefficient/1
  vel [m/s]/1 -> Sign1/1, Abs/1
  pos [m]/1 -> posFP [m]/1
  Product/1 -> F_Slide [N]/1
  sliding friction coefficient/1 -> Product/2
  Sign1/1 -> reverse/1
  FixPt Relational Operator/1 -> Stiction!/1
  Memory/1 -> FixPt Relational Operator/2
  Negative/1 -> FixPt Relational Operator/1, Memory/1
  Abs/1 -> Sum/1
  Sum/1 -> Negative/1
  Constant/1 -> Sum/2

== system nmm2DFullBody/Body Mechanics Layer (from Geyer s 2010 model)/Right Ball Contact/Ground Friction Model/X-Axis Static Friction Model ==
  note: Stiction Limit Detector
  note: Static Friction Model
  note: Zero multiplication prevents
      | horizontal friction model from
      | oscillating between static and kinetic
      | friction when the vertical force is zero but
      | the ground level is not yet reached
      | in the upward motion
  F_Normal [N] : Inport
  pos [m] : Inport  Port=2
  vel [m/s] : Inport  Port=3
  posFP [m] : Inport  Port=4
  Enable : EnablePort  StatesWhenEnabling=reset  ZeroCross=off
  Abs : Abs
  Abs. : Abs
  Check Vertical Friction : Product  RndMeth=Zero
  FixPt Relational Operator : RelationalOperator  Operator=>  OutDataTypeStr=boolean  ZeroCross=off
  Gain3 : Gain  Gain=k_gx
  Gain4 : Gain  Gain=1/v_gx_max
  Memory : Memory
  Mux1 : Mux  Inputs=2
  Positive : simulink/Logic and Bit Operations/Compare To Zero  relop=>  OutDataTypeStr=boolean
  Positive1 : simulink/Logic and Bit Operations/Compare To Zero  relop=>  OutDataTypeStr=boolean
  Sum : Sum  Inputs=-+
  Sum2 : Sum  Inputs=-+|
  X-Axis Stiction Force : Fcn  Expr=-u(1) * (1+sgn(u(1))*u(2))
  stiction limit force : Gain  Gain=mu_stick
  F_Stick [N] : Outport  OutputWhenDisabled=reset  InitialOutput=0
      settings: AttributesFormatString=when disabled: %<OutputWhenDisabled>\ninitial: %<InitialOutput>
  Sliding! : Outport  Port=2  OutputWhenDisabled=reset  InitialOutput=0
      settings: AttributesFormatString=when disabled: %<OutputWhenDisabled>\ninitial: %<InitialOutput>
  wires:
  F_Normal [N]/1 -> stiction limit force/1, Positive1/1
  Sum2/1 -> Gain3/1  "dx"
  pos [m]/1 -> Sum2/2
  posFP [m]/1 -> Sum2/1
  vel [m/s]/1 -> Gain4/1
  Sum/1 -> Positive/1
  Memory/1 -> FixPt Relational Operator/2
  Positive/1 -> FixPt Relational Operator/1, Memory/1
  Abs./1 -> Sum/2
  Mux1/1 -> X-Axis Stiction Force/1
  Gain3/1 -> Mux1/1
  Gain4/1 -> Mux1/2
  FixPt Relational Operator/1 -> Sliding!/1
  Abs/1 -> Sum/1
  stiction limit force/1 -> Abs/1
  X-Axis Stiction Force/1 -> Check Vertical Friction/1
  Positive1/1 -> Check Vertical Friction/2
  Check Vertical Friction/1 -> F_Stick [N]/1, Abs./1

== system nmm2DFullBody/Body Mechanics Layer (from Geyer s 2010 model)/Right Heel Contact/Ground Friction Model/Friction Switch ==
  note: Static/Kinetic Friction Switch
  Slide! : Inport
  Stick! : Inport  Port=2
  Memory : Memory
  S-R Flip-Flop : simulink_extras/Flip Flops/S-R Flip-Flop  initial_condition=1
  Terminator : Terminator
  Stiction : Outport
  wires:
  Memory/1 -> Stiction/1
  Slide!/1 -> S-R Flip-Flop/2
  Stick!/1 -> S-R Flip-Flop/1
  S-R Flip-Flop/2 -> Terminator/1
  S-R Flip-Flop/1 -> Memory/1

== system nmm2DFullBody/Body Mechanics Layer (from Geyer s 2010 model)/Right Heel Contact/Ground Friction Model/X-Axis Kinetic Friction Model ==
  note: Sliding Limit Detector
  note: Footpoint Determiner
  note: Kinetic Friction Model
  pos [m] : Inport
  vel [m/s] : Inport  Port=2
  F_Normal [N] : Inport  Port=3
  Enable : EnablePort  StatesWhenEnabling=reset  ZeroCross=off
  Abs : Abs
  Constant : Constant  Value=vLimit
  FixPt Relational Operator : RelationalOperator  Operator=>  OutDataTypeStr=boolean  ZeroCross=off
  Memory : Memory
  Negative : simulink/Logic and Bit Operations/Compare To Zero  relop=<  OutDataTypeStr=boolean
  Product : Product  RndMeth=Zero
  Sign1 : Signum
  Sum : Sum  Inputs=|+-
  reverse : Gain  Gain=-1
  sliding friction coefficient : Gain  Gain=mu_slide
  posFP [m] : Outport  InitialOutput=0
      settings: AttributesFormatString=initial = '%<InitialOutput>'\nwhen disabled = '%<OutputWhenDisabled>'
  Stiction! : Outport  Port=2  OutputWhenDisabled=reset  InitialOutput=0
      settings: AttributesFormatString=initial = '%<InitialOutput>'\nwhen disabled = '%<OutputWhenDisabled>'
  F_Slide [N] : Outport  Port=3  OutputWhenDisabled=reset  InitialOutput=0
      settings: AttributesFormatString=initial = '%<InitialOutput>'\nwhen disabled = '%<OutputWhenDisabled>'
  wires:
  Constant/1 -> Sum/2
  Sum/1 -> Negative/1
  Abs/1 -> Sum/1
  Negative/1 -> Memory/1, FixPt Relational Operator/1
  Memory/1 -> FixPt Relational Operator/2
  FixPt Relational Operator/1 -> Stiction!/1
  Sign1/1 -> reverse/1
  sliding friction coefficient/1 -> Product/2
  Product/1 -> F_Slide [N]/1
  pos [m]/1 -> posFP [m]/1
  vel [m/s]/1 -> Abs/1, Sign1/1
  F_Normal [N]/1 -> sliding friction coefficient/1
  reverse/1 -> Product/1

== system nmm2DFullBody/Body Mechanics Layer (from Geyer s 2010 model)/Right Heel Contact/Ground Friction Model/X-Axis Static Friction Model ==
  note: Static Friction Model
  note: Stiction Limit Detector
  note: Zero multiplication prevents
      | horizontal friction model from
      | oscillating between static and kinetic
      | friction when the vertical force is zero but
      | the ground level is not yet reached
      | in the upward motion
  F_Normal [N] : Inport
  pos [m] : Inport  Port=2
  vel [m/s] : Inport  Port=3
  posFP [m] : Inport  Port=4
  Enable : EnablePort  StatesWhenEnabling=reset  ZeroCross=off
  Abs : Abs
  Abs. : Abs
  Check Vertical Friction : Product  RndMeth=Zero
  FixPt Relational Operator : RelationalOperator  Operator=>  OutDataTypeStr=boolean  ZeroCross=off
  Gain3 : Gain  Gain=k_gx
  Gain4 : Gain  Gain=1/v_gx_max
  Memory : Memory
  Mux1 : Mux  Inputs=2
  Positive : simulink/Logic and Bit Operations/Compare To Zero  relop=>  OutDataTypeStr=boolean
  Positive1 : simulink/Logic and Bit Operations/Compare To Zero  relop=>  OutDataTypeStr=boolean
  Sum : Sum  Inputs=-+
  Sum2 : Sum  Inputs=-+|
  X-Axis Stiction Force : Fcn  Expr=-u(1) * (1+sgn(u(1))*u(2))
  stiction limit force : Gain  Gain=mu_stick
  F_Stick [N] : Outport  OutputWhenDisabled=reset  InitialOutput=0
      settings: AttributesFormatString=when disabled: %<OutputWhenDisabled>\ninitial: %<InitialOutput>
  Sliding! : Outport  Port=2  OutputWhenDisabled=reset  InitialOutput=0
      settings: AttributesFormatString=when disabled: %<OutputWhenDisabled>\ninitial: %<InitialOutput>
  wires:
  F_Normal [N]/1 -> stiction limit force/1, Positive1/1
  Sum2/1 -> Gain3/1  "dx"
  pos [m]/1 -> Sum2/2
  posFP [m]/1 -> Sum2/1
  vel [m/s]/1 -> Gain4/1
  Sum/1 -> Positive/1
  Memory/1 -> FixPt Relational Operator/2
  Positive/1 -> FixPt Relational Operator/1, Memory/1
  Abs./1 -> Sum/2
  Mux1/1 -> X-Axis Stiction Force/1
  Gain3/1 -> Mux1/1
  Gain4/1 -> Mux1/2
  FixPt Relational Operator/1 -> Sliding!/1
  Abs/1 -> Sum/1
  stiction limit force/1 -> Abs/1
  X-Axis Stiction Force/1 -> Check Vertical Friction/1
  Positive1/1 -> Check Vertical Friction/2
  Check Vertical Friction/1 -> F_Stick [N]/1, Abs./1

== system nmm2DFullBody/Full Body Control (created using the nmc library)/Left Side/AnkleJoint left/ Ankle Joint Limits ==
  note: Ankle Joint Limits
  phi [rad] : Inport
  dphi [rad/s] : Inport  Port=2
  Gain1 : Gain  Gain=c_jointstop
  Gain2 : Gain  Gain=-1
  Gain3 : Gain  Gain=c_jointstop
  Gain4 : Gain  Gain=1/w_max_jointstop
  Limit Ankle Range : simulink/Logic and Bit Operations/Interval Test  IntervalClosedRight=on  uplimit=phi12_UpLimit + 40*pi/180  IntervalClosedLeft=on  lowlimit=phi12_LowLimit - 40*pi/180  OutDataTypeStr=boolean
  Logical Operator3 : Logic  Operator=NOT  AllPortsSameDT=off  OutDataTypeStr=boolean
  Mux1 : Mux  Inputs=2
  Mux3 : Mux  Inputs=2
  Overextension Torque : Fcn  Expr="- u(1)  *  (1-u(2)) * (u(2)<1) * (u(1)>0)"
  Overflexion Torque : Fcn  Expr="- u(1)  *  (1-u(2)) * (u(2)<1) * (u(1)<0)"
  Stop Simulation1 : Stop
  Sum : Sum  Inputs=|+-
  Sum1 : Sum  Inputs=|+-
  Sum2 : Sum
  overextension angle : Constant  Value=phi12_UpLimit
  overflexion angle : Constant  Value=phi12_LowLimit
  M_stop [Nm] : Outport
  wires:
  Mux3/1 -> Overextension Torque/1
  Gain3/1 -> Mux3/1
  dphi [rad/s]/1 -> Gain4/1
  overextension angle/1 -> Sum/2
  phi [rad]/1 -> Sum/1, Sum1/1, Limit Ankle Range/1
  Sum/1 -> Gain3/1
  Gain4/1 -> Gain2/1, Mux1/2
  Gain1/1 -> Mux1/1
  Sum1/1 -> Gain1/1
  overflexion angle/1 -> Sum1/2
  Mux1/1 -> Overflexion Torque/1
  Sum2/1 -> M_stop [Nm]/1
  Gain2/1 -> Mux3/2
  Overflexion Torque/1 -> Sum2/2
  Overextension Torque/1 -> Sum2/1
  Limit Ankle Range/1 -> Logical Operator3/1
  Logical Operator3/1 -> Stop Simulation1/1

== system nmm2DFullBody/Full Body Control (created using the nmc library)/Left Side/GAS Muscle/GAS Actuation  ==
  note: GAS Actuation
  phiKnee : Inport
  phiAnkle : Inport  Port=2
  StimGas : Inport  Port=3
  " GAS" : Subsystem
  " GAS Golgi Tendon Organs" : Gain
  GAS Link : Subsystem
  GAS loop delay : TransportDelay  DelayTime=LongDelay
  Mux2 : Mux  Inputs=5
  Product2 : Product  RndMeth=Zero
  Product3 : Product  RndMeth=Zero
  Subsystem3 : nmc/Subsystem4  GotoTag=LEFT_GAS_FORCE  GotoTag2=LEFT_GAS_FORCE_LOG  GotoTag3=LEFT_GAS_FORCE_NOISE_LOG
  Subsystem5 : nmc/Subsystem4  GotoTag=LEFT_GAS_STIM  GotoTag2=LEFT_GAS_STIM_LOG  GotoTag3=LEFT_GAS_STIM_NOISE_LOG
  Subsystem6 : nmc/Subsystem4  GotoTag=LEFT_GAS_LENGTH  GotoTag2=LEFT_GAS_LENGTH_LOG  GotoTag3=LEFT_GAS_LENGTH_NOISE_LOG
  Subsystem7 : nmc/Subsystem4  GotoTag=LEFT_GAS_VELOCITY  GotoTag2=LEFT_GAS_VELOCITY_LOG  GotoTag3=LEFT_GAS_VELOCITY_NOISE_LOG
  Subsystem8 : nmc/Subsystem4  GotoTag=LEFT_GAS_GOLGI  GotoTag2=LEFT_GAS_GOLGI_LOG  GotoTag3=LEFT_GAS_GOLGI_NOISE_LOG
  Terminator2 : Terminator
  TauGasKnee : Outport
  TauGasAnkle : Outport  Port=2
  FmGas : Outport  Port=3
  wires:
  " GAS"/1(Fmtc) -> Subsystem3/1
  GAS Link/3(lever12 [m]) -> Product2/2
  GAS Link/2(lever23 [m]) -> Product3/2
  GAS Link/1(lmtu [m]) -> " GAS"/2(lmtc [m])
  Product3/1 -> TauGasKnee/1
  " GAS"/5(A) -> Mux2/5
  Mux2/1 -> Terminator2/1
  " GAS"/4(Lse) -> Mux2/4
  " GAS"/3(Vce) -> Subsystem7/1
  " GAS"/2(Lce) -> Subsystem6/1
  phiKnee/1 -> GAS Link/1(phi23 [rad])
  phiAnkle/1 -> GAS Link/2(phi12 [rad])
  StimGas/1 -> Subsystem5/1
  Product2/1 -> TauGasAnkle/1
  " GAS Golgi Tendon Organs"/1 -> GAS loop delay/1
  GAS loop delay/1 -> FmGas/1
  Subsystem5/1 -> " GAS"/1(STIM)
  Subsystem3/1 -> Mux2/1, Product2/1, Product3/1, Subsystem8/1
  Subsystem6/1 -> Mux2/2
  Subsystem7/1 -> Mux2/3
  Subsystem8/1 -> " GAS Golgi Tendon Organs"/1

== system nmm2DFullBody/Full Body Control (created using the nmc library)/Left Side/GAS Muscle/GAS Control ==
  note: GAS sControl
  FmGAS : Inport
  StanceSwing : Inport  Port=2
  " Swing Phase" : Subsystem  TreatAsAtomicUnit=on
  "ANMC STIM " : Concatenate  NumInputs=1
  Logical Operator : Logic  Operator=NOT  AllPortsSameDT=off  OutDataTypeStr=boolean
  Saturation17 : Saturate  UpperLimit=1  LowerLimit=0.01  ZeroCross=off
  Stance Phase : Subsystem  TreatAsAtomicUnit=on
  Sum18 : Sum
  StimGAS : Outport
  wires:
  Logical Operator/1 -> " Swing Phase"/Enable
  FmGAS/1 -> Stance Phase/1(FmGAS)
  StanceSwing/1 -> Logical Operator/1, Stance Phase/Enable
  " Swing Phase"/1(StimGAS) -> Sum18/2
  Sum18/1 -> Saturation17/1
  Saturation17/1 -> "ANMC STIM "/1
  Stance Phase/1(StimGAS) -> Sum18/1
  "ANMC STIM "/1 -> StimGAS/1

== system nmm2DFullBody/Full Body Control (created using the nmc library)/Left Side/GLU Muscle/GLU Actuation ==
  note: GLU Actuation
  phiHip : Inport
  StimGlu : Inport  Port=2
  " GLU" : Subsystem
  " GLU Fm loop delay" : TransportDelay  DelayTime=ShortDelay
  GLU Golgi Tendon Organs : Gain
  GLU Link : Subsystem
  Mux : Mux  Inputs=5
  Product6 : Product  RndMeth=Zero
  Subsystem3 : nmc/Subsystem4  GotoTag=LEFT_GLU_FORCE  GotoTag2=LEFT_GLU_FORCE_LOG  GotoTag3=LEFT_GLU_FORCE_NOISE_LOG
  Subsystem5 : nmc/Subsystem4  GotoTag=LEFT_GLU_STIM  GotoTag2=LEFT_GLU_STIM_LOG  GotoTag3=LEFT_GLU_STIM_NOISE_LOG
  Subsystem6 : nmc/Subsystem4  GotoTag=LEFT_GLU_LENGTH  GotoTag2=LEFT_GLU_LENGTH_LOG  GotoTag3=LEFT_GLU_LENGTH_NOISE_LOG
  Subsystem7 : nmc/Subsystem4  GotoTag=LEFT_GLU_VELOCITY  GotoTag2=LEFT_GLU_VELOCITY_LOG  GotoTag3=LEFT_GLU_VELOCITY_NOISE_LOG
  Subsystem8 : nmc/Subsystem4  GotoTag=LEFT_GLU_GOLGI  GotoTag2=LEFT_GLU_GOLGI_LOG  GotoTag3=LEFT_GLU_GOLGI_NOISE_LOG
  Terminator : Terminator
  TauGlu : Outport
  FmGlu : Outport  Port=2
  wires:
  " GLU"/1(Fmtc) -> Subsystem3/1
  StimGlu/1 -> Subsystem5/1
  Product6/1 -> TauGlu/1
  GLU Link/1(lmtu [m]) -> " GLU"/2(lmtc [m])
  GLU Link/2(lever [m]) -> Product6/2
  " GLU"/5(A) -> Mux/5
  GLU Golgi Tendon Organs/1 -> " GLU Fm loop delay"/1
  " GLU"/2(Lce) -> Subsystem6/1
  " GLU"/3(Vce) -> Subsystem7/1
  " GLU"/4(Lse) -> Mux/4
  Mux/1 -> Terminator/1
  phiHip/1 -> GLU Link/1(phi34 [rad])
  " GLU Fm loop delay"/1 -> FmGlu/1
  Subsystem6/1 -> Mux/2
  Subsystem7/1 -> Mux/3
  Subsystem5/1 -> " GLU"/1(STIM)
  Subsystem3/1 -> Mux/1, Subsystem8/1, Product6/1
  Subsystem8/1 -> GLU Golgi Tendon Organs/1

== system nmm2DFullBody/Full Body Control (created using the nmc library)/Left Side/GLU Muscle/GLU Control ==
  note: GLU Control
  FmGlu : Inport
  Theta : Inport  Port=2
  dTheta : Inport  Port=3
  CLdxThigh : Inport  Port=4
  OLonCL : Inport  Port=5
  StanceSwing : Inport  Port=6
  " Swing Phase" : Subsystem  TreatAsAtomicUnit=on
  "ANMC STIM " : Concatenate  NumInputs=1
  Logical Operator : Logic  Operator=NOT  AllPortsSameDT=off  OutDataTypeStr=boolean
  Saturation17 : Saturate  UpperLimit=1  LowerLimit=0.01  ZeroCross=off
  Stance Phase : Subsystem  TreatAsAtomicUnit=on
  Sum18 : Sum
  StimGlu : Outport
  wires:
  Logical Operator/1 -> " Swing Phase"/Enable
  " Swing Phase"/1(StimGLU) -> Sum18/2
  FmGlu/1 -> " Swing Phase"/1(FmGLU)
  Sum18/1 -> Saturation17/1
  Saturation17/1 -> "ANMC STIM "/1
  dTheta/1 -> Stance Phase/2(dTheta [rad/s])
  Theta/1 -> Stance Phase/1(Theta)
  Stance Phase/1(StimGLU) -> Sum18/1
  CLdxThigh/1 -> Stance Phase/3(CLdxThigh [N])
  OLonCL/1 -> Stance Phase/4(OLonCL)
  StanceSwing/1 -> Logical Operator/1, Stance Phase/Enable
  "ANMC STIM "/1 -> StimGlu/1
